simulink model "tst_bus2_BUG"  (Simulink 8.0)
settings: Solver=ode45  StartTime=0.0  StopTime=10.0  RelTol=1e-3
settings Model: Creator=Marci  LastModifiedBy=Marci

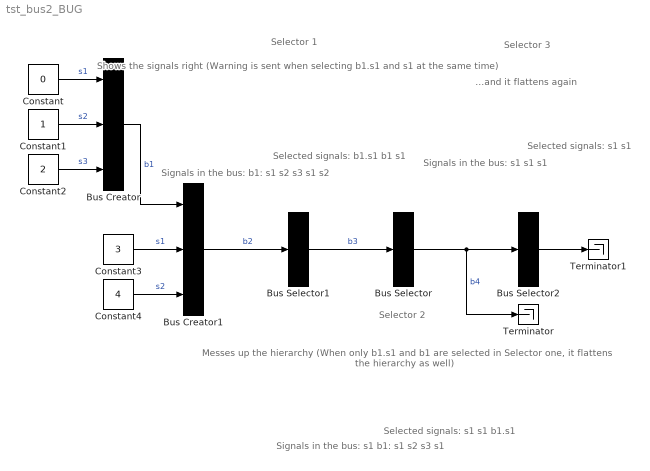
== system tst_bus2_BUG ==
  note: Selected signals:
      | b1.s1
      | b1
      | s1
  note: Signals in the bus:
      | b1:
      | 	s1
      | 	s2
      | 	s3
      | s1
      | s2
  note: ...and it flattens again
  note: Messes up the hierarchy
      | (When only b1.s1 and b1 are
      | selected in Selector one,
      | it flattens the hierarchy as well)
  note: Shows the signals right
      | (Warning is sent when selecting
      | b1.s1 and s1 at the same time)
  note: Selector 3
  note: Selector 1
  note: Selector 2
  note: Selected signals:
      | s1
      | s1
      | b1.s1
  note: Signals in the bus:
      | s1
      | b1:
      | 	s1
      | 	s2
      | 	s3
      | s1
  note: Selected signals:
      | s1
      | s1
  note: Signals in the bus:
      | s1
      | s1
      | s1
  Bus Creator : BusCreator  Inputs=3
  Bus Creator1 : BusCreator  Inputs=3
  Bus Selector : BusSelector  OutputSignals=s1,s1,b1.s1  OutputAsBus=on
  Bus Selector1 : BusSelector  OutputSignals=b1.s1,b1,s1  OutputAsBus=on
  Bus Selector2 : BusSelector  OutputSignals=s1,s1  OutputAsBus=on
  Constant : Constant  Value=0
  Constant1 : Constant
  Constant2 : Constant  Value=2
  Constant3 : Constant  Value=3
  Constant4 : Constant  Value=4
  Terminator : Terminator
  Terminator1 : Terminator
  wires:
  Bus Creator/1 -> Bus Creator1/1  "b1"
  Constant/1 -> Bus Creator/1  "s1"
  Constant1/1 -> Bus Creator/2  "s2"
  Constant2/1 -> Bus Creator/3  "s3"
  Constant3/1 -> Bus Creator1/2  "s1"
  Constant4/1 -> Bus Creator1/3  "s2"
  Bus Creator1/1 -> Bus Selector1/1  "b2"
  Bus Selector/1 -> Bus Selector2/1, Terminator/1  "b4"
  Bus Selector1/1 -> Bus Selector/1  "b3"
  Bus Selector2/1 -> Terminator1/1
